simulink model "uGrid_1PH_hd_ATD_prueba"  (R2018a)
settings: Solver=ode45  StartTime=0.0  StopTime=1.5  FixedStep=1e-4  MaxStep=1e-4  RelTol=1e-3
PreLoadFcn:
  | SimulinkInit
InitFcn:
  | SimulinkInit
values from neighbouring files (symbols this model uses):
  Ad = sysd.A    [SimulinkInit.m]
  b = 4.91    [parametros_BIO.m]
  Bd = sysd.B    [SimulinkInit.m]
  C = C1+C2+C3+Cl    (= 0.002654)    [SimulinkInit.m]    (also in parametros_BIO.m = 1)
  C1 = Cd(1,:)    [SimulinkInit.m]
  C2 = Cd(2,:)    [SimulinkInit.m]
  C3 = Cd(3,:)    [SimulinkInit.m]
  C4 = Cd(4,:)    [SimulinkInit.m]
  Cd = sysd.C    [SimulinkInit.m]
  K = 25    [parametros_BIO.m]    (also in uio_linear.m = K1+E*H)
  K1 = 1.15    [SimulinkInit.m]    (also in parametros_BIO.m = 9.66; uio_linear.m = K1')
  K11 = 0.8    [parametros_BIO.m]
  K2 = 1    [SimulinkInit.m]    (also in parametros_BIO.m = 6.97)
  K22 = 0.2    [parametros_BIO.m]
  K3 = 1    [SimulinkInit.m]    (also in parametros_BIO.m = 31.8)
  K33 = 0.23    [parametros_BIO.m]
  K4 = 15.1    [parametros_BIO.m]
  Kd = 0.02    [parametros_BIO.m]
  Kdc = 0.02    [parametros_BIO.m]
  Kf = 1    [parametros_BIO.m]
  Kh = 1.2    [parametros_BIO.m]
  Ks = 21.5    [parametros_BIO.m]
  Ksc = 3    [parametros_BIO.m]
  Kv = 1    [parametros_BIO.m]
  Sbin = 13.8    [parametros_BIO.m]
  Svin = 2.91    [parametros_BIO.m]
  T1 = 0.4    [parametros_BIO.m]
  T2 = 1    [parametros_BIO.m]
  T3 = 15    [parametros_BIO.m]
  T4 = 2.5    [parametros_BIO.m]
  T5 = 3.3    [parametros_BIO.m]
  Tao1 = 0.5    [SimulinkInit.m]
  Tcd = 0.2    [parametros_BIO.m]
  Tcr = 0.01    [parametros_BIO.m]
  Tf = 0.04    [parametros_BIO.m]
  tm = 1e-4    (= 0.0001)    [SimulinkInit.m]
  Tr = 950    [parametros_BIO.m]
  Tt = 450    [parametros_BIO.m]
  Ttd = 0.04    [parametros_BIO.m]
  Tv = 0.05    [parametros_BIO.m]
  V = 20    [parametros_BIO.m]
  wref = 70000    [parametros_BIO.m]
  X_acid = 1.2    [parametros_BIO.m]
  X_meth = 0.35    [parametros_BIO.m]
  Z = 3    [parametros_BIO.m]
undefined symbols (not defined in the file or in its folder): F1, F2, F3, F4, G, GF, H1, H2, H3, H4, Ion, K1U, K2U, K3U, K4U, Lithium, ss1, ss2
libraries: powerlib x58, dsparch4 x12, truetime x12, powerlib_meascontrol x4, simulink x1, electricdrivelib x1
(part 1 of 3)
settings Model: Creator=erich  LastModifiedBy=carma
settings CodeAppCC: StateflowObjectComments=on
settings SimscapeCC: SimscapeNormalizeSystem=off

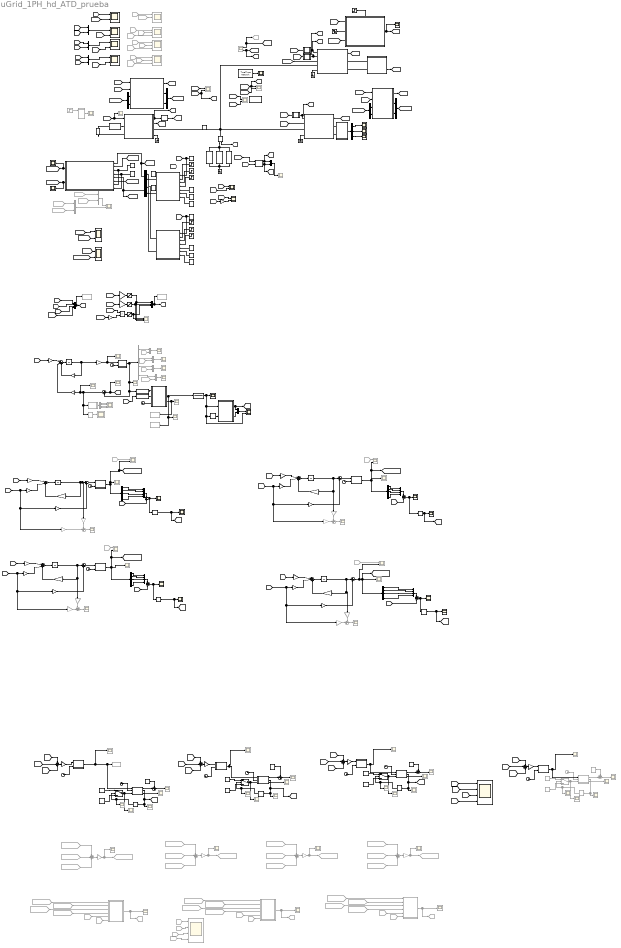
== system uGrid_1PH_hd_ATD_prueba ==
  note: DIESEL VSI
  note: Load
  note: BIO - CSI
  note: RENEWABLE - CSI
  note: Nodo De Optimizacion
  1Ph_Inverter_bio : Subsystem  mask{st_time=0, f_sw=12000, samp_f=1e-6}
      mask prompts: st_time "Tiempo muerto (Start)"; f_sw "Switching frequency"; samp_f "samplig"
      mask Display:
      | port_label('input', 1, 'd', 'texmode', 'on')
      | 
      | port_label('lconn', 1, 'DC +')
      | port_label('lconn', 2, 'DC -')
      | 
      | 
      | port_label('rconn', 1, 'V_{out+}')
      | port_label('rconn', 2, 'B_{out-}')
      | 
      | 
      | port_label('output', 1, 'I_{out}', 'texmode', 'on')
      | port_label('output', 2, 'V_{out}', 'texmode', 'on')
      | 
      | plot([0.1 .9], [0.1 .9])
      | plot([0.2 .4], [.7 .7])
      | plot([0.2 .24], [.65 .65])
      | plot([0.28 .32], [.65 .65])
      | plot([0.36 .40], [.65 .65])
      | 
      | plot([.5:.01:.7], .25+sin(30*[.2:.01:.4])/10)
  1Ph_Inverter_bio1 : Subsystem  mask{st_time=0, f_sw=12000, samp_f=1e-6}
      mask prompts: st_time "Tiempo muerto (Start)"; f_sw "Switching frequency"; samp_f "samplig"
      mask Display:
      | port_label('input', 1, 'd', 'texmode', 'on')
      | 
      | port_label('lconn', 1, 'DC +')
      | port_label('lconn', 2, 'DC -')
      | 
      | 
      | port_label('rconn', 1, 'V_{out+}')
      | port_label('rconn', 2, 'B_{out-}')
      | 
      | 
      | port_label('output', 1, 'I_{out}', 'texmode', 'on')
      | port_label('output', 2, 'V_{out}', 'texmode', 'on')
      | port_label('output', 3, 'I_{cap}', 'texmode', 'on')
      | 
      | plot([0.1 .9], [0.1 .9])
      | plot([0.2 .4], [.7 .7])
      | plot([0.2 .24], [.65 .65])
      | plot([0.28 .32], [.65 .65])
      | plot([0.36 .40], [.65 .65])
      | 
      | plot([.5:.01:.7], .25+sin(30*[.2:.01:.4])/10)
  1Ph_Inverter_diesel : Subsystem  mask{st_time=0, f_sw=12000, samp_f=1e-6}
      mask prompts: st_time "Tiempo muerto (Start)"; f_sw "Switching frequency"; samp_f "Sampling frequency"
      mask Display:
      | port_label('input', 1, 'd', 'texmode', 'on')
      | 
      | port_label('lconn', 1, 'DC +')
      | port_label('lconn', 2, 'DC -')
      | 
      | 
      | port_label('rconn', 1, 'V_{out+}')
      | port_label('rconn', 2, 'B_{out-}')
      | 
      | 
      | port_label('output', 1, 'I_{out}', 'texmode', 'on')
      | port_label('output', 2, 'V_{out}', 'texmode', 'on')
      | 
      | plot([0.1 .9], [0.1 .9])
      | plot([0.2 .4], [.7 .7])
      | plot([0.2 .24], [.65 .65])
      | plot([0.28 .32], [.65 .65])
      | plot([0.36 .40], [.65 .65])
      | 
      | plot([.5:.01:.7], .25+sin(30*[.2:.01:.4])/10)
  Bus Selector : BusSelector  OutputSignals=SOC (%),Current (A),Voltage (V)
  CSI_Control_BIO : Subsystem
  CSI_Control_DIESEL : Subsystem
  Clock{,1..5,14,18..22} (12 alike) : Clock
  Clock15 : Clock  Commented=on
  Constant : Constant  Value=1000
  Constant{1,4..5,7} (4 alike) : Constant  Value=4000
  Constant{9..11,13..14,16} (6 alike) : Constant
  Constant12 : Constant  Value=0
  Constant15 : Constant  Value=0
  Constant17 : Constant  Commented=on
  Constant18 : Constant  Commented=on  Value=0
  Constant19 : Constant  Commented=on
  Constant2 : Constant  Value=11210
  Constant3 : Constant  Value=5000
  Constant6 : Constant  Value=5000
  Constant8 : Constant  Value=0
  DC 1000V : powerlib/Electrical Sources/DC Voltage Source  Amplitude=1000  Measurements=None
  DIESEL + Rectifier System : Subsystem
  Delay2 : Delay  DelayLength=1
  Demux : Demux  Outputs=2
  Demux1 : Demux  Outputs=2
  Demux19 : Demux  Commented=on
  Demux2 : Demux  Commented=on
  Demux{5..8} (4 alike) : Demux  Outputs=5
  Derivative{,1..2,4} (4 alike) : Derivative  CoefficientInTFapproximation=0
  Derivative3 : Derivative  Commented=on  CoefficientInTFapproximation=0
  DynMat : Constant  Value=G
  DynMat_RespLibre : Constant  Value=GF
  From100 : From  Commented=on  GotoTag=x_hat_uio3
  From101 : From  Commented=on  GotoTag=x_hat_uio4
  From116 : From  Commented=on  GotoTag=x_hat_uio1
  From117 : From  Commented=on  GotoTag=rol
  From118 : From  Commented=on  GotoTag=ruo1
  From119 : From  Commented=on  GotoTag=x_hat_uio21
  From120 : From  Commented=on  GotoTag=x_hat_uio22
  From121 : From  Commented=on  GotoTag=x_hat_uio23
  From122 : From  Commented=on  GotoTag=x_hat_uio2
  From123 : From  Commented=on  GotoTag=x_hat_uio31
  From124 : From  Commented=on  GotoTag=x_hat_uio32
  From125 : From  Commented=on  GotoTag=x_hat_uio33
  From126 : From  Commented=on  GotoTag=x_hat_uio41
  From127 : From  Commented=on  GotoTag=x_hat_uio42
  From128 : From  Commented=on  GotoTag=x_hat_uio43
  From129 : From  Commented=on  GotoTag=x_hat_uio3
  From130 : From  Commented=on  GotoTag=x_hat_uio4
  From131 : From  Commented=on  GotoTag=x_hat_uio1
  From132 : From  Commented=on  GotoTag=rol
  From133 : From  Commented=on  GotoTag=ruo2
  From134 : From  Commented=on  GotoTag=x_hat_uio2
  From135 : From  Commented=on  GotoTag=x_hat_uio3
  From136 : From  Commented=on  GotoTag=x_hat_uio4
  From137 : From  Commented=on  GotoTag=x_hat_uio1
  From138 : From  Commented=on  GotoTag=rol
  From139 : From  Commented=on  GotoTag=ruo3
  From140 : From  Commented=on  GotoTag=x_hat_uio2
  From143 : From  Commented=on  GotoTag=ca4
  From144 : From  Commented=on  GotoTag=ca3
  From145 : From  Commented=on  GotoTag=ca2
  From148 : From  Commented=on  GotoTag=ca1
  From150 : From  Commented=on  GotoTag=V_vsi
  From153 : From  Commented=on  GotoTag=I3
  From154 : From  Commented=on  GotoTag=I2
  From155 : From  Commented=on  GotoTag=I1
  From159 : From  Commented=on  GotoTag=I1r
  From160 : From  Commented=on  GotoTag=I2r
  From162 : From  Commented=on  GotoTag=I3r
  From163 : From  Commented=on  GotoTag=Vlreal
  From165 : From  Commented=on  GotoTag=ruo3
  From166 : From  Commented=on  GotoTag=ruo1
  From167 : From  Commented=on  GotoTag=ruo2
  From20 : From  Commented=on  GotoTag=set_BIO
  From21 : From  Commented=on  GotoTag=set_DIESEL
  From22 : From  Commented=on  GotoTag=PQ_meas_diesel
  From23 : From  Commented=on  GotoTag=PQ_meas_bio
  From{26,58,64..65} (4 alike) : From  Commented=on  GotoTag=y_ma
  From76 : From  Commented=on  GotoTag=I1
  From77 : From  Commented=on  GotoTag=I2
  From78 : From  Commented=on  GotoTag=I3
  From79 : From  Commented=on  GotoTag=V_vsi
  From97 : From  Commented=on  GotoTag=x_hat_uio11
  From98 : From  Commented=on  GotoTag=x_hat_uio12
  From99 : From  Commented=on  GotoTag=x_hat_uio13
  Gain{,1,3,7} (4 alike) : Gain  Gain=1/3
  Gain{8..11} (4 alike) : Gain  Commented=on  Gain=1/3
  Gain2 : Gain  Gain=-1
  Gain4 : Gain  Gain=2000
  Gain5 : Gain  Gain=2
  Gain6 : Gain  Gain=2000
  Goto16 : Goto  Commented=on  GotoTag=Vlreal
  Goto24 : Goto  Commented=on  GotoTag=ca1
  Goto40 : Goto  Commented=on  GotoTag=x_hat_uio1
  Goto42 : Goto  Commented=on  GotoTag=x_hat_uio2
  Goto43 : Goto  Commented=on  GotoTag=x_hat_uio3
  Goto44 : Goto  Commented=on  GotoTag=x_hat_uio4
  Goto61 : Goto  Commented=on  GotoTag=ca2
  Goto62 : Goto  Commented=on  GotoTag=ca3
  Ground{,1..3} (4 alike) : powerlib/Elements/Ground  LConnTagsString=a
  I sens A : powerlib/Measurements/Current Measurement  PhasorSimulation=off  OutputType=Complex  PSBequivalent=0
  LinearProg : MATLAB Function  TreatAsAtomicUnit=on  SystemSampleTime=1e-3
  LinearProg1 : MATLAB Function  TreatAsAtomicUnit=on  SystemSampleTime=1e-3
  MATLAB Function : MATLAB Function  TreatAsAtomicUnit=on
  MATLAB Function1 : MATLAB Function  TreatAsAtomicUnit=on
  MATLAB Function10 : MATLAB Function  TreatAsAtomicUnit=on
  MATLAB Function11 : MATLAB Function  TreatAsAtomicUnit=on
  MATLAB Function14 : MATLAB Function  Commented=on  TreatAsAtomicUnit=on
  MATLAB Function2 : MATLAB Function  Commented=on  TreatAsAtomicUnit=on
  MATLAB Function23 : MATLAB Function  TreatAsAtomicUnit=on
  MATLAB Function24 : MATLAB Function  TreatAsAtomicUnit=on
  MATLAB Function25 : MATLAB Function  TreatAsAtomicUnit=on
  MATLAB Function3 : MATLAB Function  TreatAsAtomicUnit=on
  MATLAB Function34 : MATLAB Function  Commented=on  TreatAsAtomicUnit=on
  MATLAB Function36 : MATLAB Function  TreatAsAtomicUnit=on
  MATLAB Function38 : MATLAB Function  Commented=on  TreatAsAtomicUnit=on
  MATLAB Function39 : MATLAB Function  Commented=on  TreatAsAtomicUnit=on
  MATLAB Function4 : MATLAB Function  TreatAsAtomicUnit=on
  MATLAB Function5 : MATLAB Function  TreatAsAtomicUnit=on
  MATLAB Function6 : MATLAB Function  TreatAsAtomicUnit=on
  MATLAB Function7 : MATLAB Function  TreatAsAtomicUnit=on
  MPC Controller : Subsystem
  MeasureNode_I1 : Subsystem
  MeasureNode_I2 : Subsystem
  MeasureNode_I3 : Subsystem
  MeasureNode_I4 : Subsystem
  Memory : Memory
  Memory1 : Memory
  Memory2 : Memory
  Memory3 : Memory  Commented=on
  Mux{,1,4..6,14,26..28} (9 alike) : Mux  Inputs=2
  Mux{2..3,9..12} (6 alike) : Mux  Commented=on  Inputs=2
  Mux{8,16..19} (5 alike) : Mux
  Mux7 : Mux  Inputs=3
  P_lp_bio : Constant  Value=500
  P_lp_diesel : Constant  Value=300
  Power : powerlib_meascontrol/Measurements/Power  Freq=60  Vinit=[1, 0]  Iinit=[1, 0]  Ts=0
      settings: SourceProductName=Simscape Power Systems
  Product1 : Product
  RL : powerlib/Elements/Series RLC Branch  LConnTagsString=__new0  RConnTagsString=__new0  BranchType=R  Resistance=10  Inductance=500e-3  SetiL0=off  InitialCurrent=0  Capacitance=100e-6  Setx0=off  InitialVoltage=0  Measurements=None
  RL1 : powerlib/Elements/Series RLC Branch  LConnTagsString=__new0  RConnTagsString=__new0  BranchType=RL  Resistance=10  Inductance=5.2  SetiL0=off  InitialCurrent=0  Capacitance=100e-6  Setx0=off  InitialVoltage=0  Measurements=None
  RL2 : powerlib/Elements/Series RLC Branch  LConnTagsString=__new0  RConnTagsString=__new0  BranchType=C  Resistance=30  Inductance=500e-3  SetiL0=off  InitialCurrent=0  Capacitance=2000e-6  Setx0=off  InitialVoltage=0  Measurements=None
  Rin : powerlib/Elements/Series RLC Branch  LConnTagsString=__new0  RConnTagsString=__new0  BranchType=R  Resistance=.001  Inductance=0  SetiL0=off  InitialCurrent=0  Capacitance=0  Setx0=off  InitialVoltage=0  Measurements=None
  Saturation3 : Saturate  UpperLimit=1000  LowerLimit=-1000
  Saturation4 : Saturate  UpperLimit=1000  LowerLimit=-1000
  Saturation5 : Saturate  UpperLimit=1000  LowerLimit=-1000
  Scope{,1..3,7,85..88} (9 alike) : Scope  Commented=on  NumInputPorts=2
  Scope{5..6,9..13,41,49..50,55,64,106,111,113,115} (16 alike) : Scope
  Scope{4,8,23,31..40,45,48,51,53,57..58,60..63,67,98..99,105,107..110,112,114,118,120..138} (53 alike) : Scope  Commented=on
  Scope15 : Scope  Commented=on  NumInputPorts=4
  Scope19 : Scope  NumInputPorts=4
  Scope{24..25,27..28,42,52,59,66,73} (9 alike) : Scope  NumInputPorts=2
  Scope{30,46,56,65,68} (5 alike) : Scope  Commented=on  NumInputPorts=3
  Scope43 : Scope  Commented=on  NumInputPorts=4
  Signal Specification : SignalSpecification  Dimensions=4
  Signal Specification1 : SignalSpecification  Dimensions=4
  Sine Wave : Sin  Amplitude=170  Frequency=2*pi*60  SampleTime=0
  Step : Step  Commented=on  Time=0  After=28  SampleTime=0
  Step1 : Step  Time=0.3  Before=20000  After=5000  SampleTime=0
  Step2 : Step  Time=.6  Before=1.2  After=.4  SampleTime=0
  Step3 : Step  Before=.7  After=.7  SampleTime=0
  Step4 : Step  Time=10e-3  SampleTime=0
  Step5 : Step  Time=.3  Before=20000  After=5000  SampleTime=0
  Step6 : Step  Time=.6  Before=1.2  After=.4  SampleTime=0
  Step7 : Step  Before=.7  After=.7  SampleTime=0
  Subsystem : Subsystem
  Sum{,3,7,15} (4 alike) : Sum  Inputs=|++
  Sum{1..2,5,11} (4 alike) : Sum  Inputs=+-
  Sum10 : Sum  Inputs=|+-
  Sum{6,12,23..24} (4 alike) : Sum  Commented=on  Inputs=-+|
  Sum{4,8..9,14,16} (5 alike) : Sum  Inputs=|+++  SampleTime=tm
  Sum{50..52,56} (4 alike) : Sum  Inputs=+++
  Sum53 : Sum  Inputs=+-|
  Sum54 : Sum  Inputs=+-|
  Sum55 : Sum  Inputs=+-|
  Sum57 : Sum  Commented=on  Inputs=+-|
  Sum{58..61} (4 alike) : Sum  Commented=on  Inputs=+++
  Switch : Switch  Criteria=u2 > Threshold
  Switch1 : Switch  Criteria=u2 > Threshold
  Switch2 : Switch  Criteria=u2 > Threshold
  Switch3 : Switch  Commented=on  Criteria=u2 > Threshold
  To Workspace : ToWorkspace  Commented=on  VariableName=det1  SampleTime=1e-4
  To Workspace1 : ToWorkspace  Commented=on  VariableName=norm1  SampleTime=1e-4
  To Workspace2 : ToWorkspace  Commented=on  VariableName=y_ma  SampleTime=1e-4
  To Workspace3 : ToWorkspace  Commented=on  VariableName=u_fs  SampleTime=1e-4
  To Workspace4 : ToWorkspace  Commented=on  VariableName=dr  SaveFormat=Structure With Time  SampleTime=-1
  Transfer Fcn6 : TransferFcn  Denominator=[0.005 1]
  TrueTime Network : truetime/TrueTime Network  nwtype=CSMA/CD (Ethernet)  nwnbr=1  nnodes=10  rate=8*1e9  minsize=512  lossprob=0  seed=0  bandwidths=[0.5 0.5]  slotsize=512  schedule=[1 1 2]  memsize=80000  buftype=Common buffer  overflow=Retransmit  dynSchedule=0  miniSlotSize=0  NIT=0  QSortMode=FIFO  sync=0  irtSchedule=0  nrtLength=0  nodeGraph=0  scheduleoutput=on
  Unit Delay{1..2,6..7,10} (5 alike) : UnitDelay  SampleTime=tm
  VSI_Controller : Subsystem
  adis1 : Gain  Gain=F3  Multiplication=Matrix(K*u) (u vector)  SampleTime=tm
  adis10 : Gain  Gain=Ld'  Multiplication=Matrix(K*u) (u vector)  SampleTime=tm
  adis11 : Gain  Gain=F1  Multiplication=Matrix(K*u) (u vector)  SampleTime=tm
  adis12 : Gain  Gain=F2  Multiplication=Matrix(K*u) (u vector)  SampleTime=tm
  adis2 : Gain  Gain=F4  Multiplication=Matrix(K*u) (u vector)  SampleTime=tm
  adis7 : Gain  Gain=Ad  Multiplication=Matrix(K*u) (u vector)  SampleTime=tm
  bdis1 : Gain  Gain=T3*Bd  Multiplication=Matrix(K*u) (u vector)  SampleTime=tm
  bdis10 : Gain  Gain=T2*Bd  Multiplication=Matrix(K*u) (u vector)  SampleTime=tm
  bdis11 : Gain  Gain=K2U  Multiplication=Matrix(K*u) (u vector)  SampleTime=tm
  bdis12 : Gain  Gain=H2  Multiplication=Matrix(K*u) (u vector)  SampleTime=tm
  bdis13 : Gain  Commented=on  Gain=eye(1)-C2*H2  Multiplication=Matrix(K*u) (u vector)  SampleTime=tm
  bdis14 : Gain  Commented=on  Gain=eye(1)-C1*H1  Multiplication=Matrix(K*u) (u vector)  SampleTime=tm
  bdis15 : Gain  Commented=on  Gain=C1  Multiplication=Matrix(K*u) (u vector)  SampleTime=tm
  bdis16 : Gain  Commented=on  Gain=C2  Multiplication=Matrix(K*u) (u vector)  SampleTime=tm
  bdis17 : Gain  Gain=T4*Bd  Multiplication=Matrix(K*u) (u vector)  SampleTime=tm
  bdis18 : Gain  Gain=K4U  Multiplication=Matrix(K*u) (u vector)  SampleTime=tm
  bdis19 : Gain  Gain=H4  Multiplication=Matrix(K*u) (u vector)  SampleTime=tm
  bdis2 : Gain  Gain=K3U  Multiplication=Matrix(K*u) (u vector)  SampleTime=tm
  bdis20 : Gain  Commented=on  Gain=eye(1)-C4*H4  Multiplication=Matrix(K*u) (u vector)  SampleTime=tm
  bdis21 : Gain  Commented=on  Gain=C4  Multiplication=Matrix(K*u) (u vector)  SampleTime=tm
  bdis3 : Gain  Gain=H3  Multiplication=Matrix(K*u) (u vector)  SampleTime=tm
  bdis4 : Gain  Commented=on  Gain=eye(1)-C3*H3  Multiplication=Matrix(K*u) (u vector)  SampleTime=tm
  bdis5 : Gain  Gain=Bd  Multiplication=Matrix(K*u) (u vector)  SampleTime=tm
  bdis6 : Gain  Commented=on  Gain=C3  Multiplication=Matrix(K*u) (u vector)  SampleTime=tm
  bdis7 : Gain  Gain=T1*Bd  Multiplication=Matrix(K*u) (u vector)  SampleTime=tm
  bdis8 : Gain  Gain=K1U  Multiplication=Matrix(K*u) (u vector)  SampleTime=tm
  bdis9 : Gain  Gain=H1  Multiplication=Matrix(K*u) (u vector)  SampleTime=tm
  cdis4 : Gain  Gain=Cd  Multiplication=Matrix(K*u) (u vector)  SampleTime=tm
  generador biomasa : Subsystem  Commented=on
  powergui : powerlib/powergui  Priority=1  SimulationMode=Continuous  SampleTime=50e-6  frequency=60  Iterations=50  frequencyindice=0  Pbase=100e6  ErrMax=1e-4  UnitsV=kV  UnitsW=MW  buscounter=0  FunctionMessages=off  echomessages=off  EnableUseOfTLC=off  CurrentSourceSwitches=off  DisableSnubberDevices=off  DisableRonSwitches=off  DisableVfSwitches=off  DisplayEquations=off  SolverType=Tustin/Backward Euler (TBE)  Interpol=off  ExternalGateDelay=off  methode=off  Ts=100  x0status=blocks  SPID=off  SwTol=0  HookPort=off  RestoreLinks=warning  ResistiveCurrentMeasurement=off  Frange=[0:2:500]  Ylog=off  Xlog=on  ShowGrid=off  save=off  variable=ZData  structure=0  ZoomFFT=off  StartTime=0.0  cycles=1  DisplayStyle=1  fundamental=60  FreqAxis=off  MaxFrequency=1000  frequencyindicesteady=1  RmsSteady=1  display=off
  1000 : Constant  IOType=siggen
  wires:
  [D_bio] -> Scope4/1, 1Ph_Inverter_bio/1(A_in)
  [D_die] -> 1Ph_Inverter_diesel/1(A_in)
  [I_bio] -> [I1], Scope2/2
  [V_bio] -> Scope2/1
  [I_die] -> [I2], Scope3/1
  [V_die] -> Scope3/2
  1Ph_Inverter_bio/1(Iout) -> [I1r], MeasureNode_I2/1(in)
  1Ph_Inverter_bio/2(Vout) -> [V_bio]
  1Ph_Inverter_diesel/1(Iout) -> [I2r], MeasureNode_I1/1(in)
  1Ph_Inverter_diesel/2(Vout) -> [V_die]
  CSI_Control_BIO/1(D) -> [D_bio]
  [I_bio] -> CSI_Control_BIO/2(I_measured)
  [V_bio] -> CSI_Control_BIO/1(V_measured)
  CSI_Control_DIESEL/1(D) -> [D_die]
  [I_die] -> CSI_Control_DIESEL/2(I_measured)
  [V_die] -> CSI_Control_DIESEL/1(V_measured)
  [I_vsi] -> Scope1/1
  [I_load] -> Scope1/2
  Mux/1 -> [PQ_meas_bio]
  [MPC_U_bio] -> Demux/1
  [MPC_U_diesel] -> Demux1/1
  Mux1/1 -> [PQ_meas_diesel]
  From21/1 -> Mux2/2  "set_DIESEL"
  From20/1 -> Mux2/1  "set_BIO"
  Mux2/1 -> Scope/1
  Mux3/1 -> Scope/2
  From22/1 -> Mux3/2  "meas_DIESEL"
  From23/1 -> Mux3/1  "meas_BIO"
  CSI_Control_BIO/2(P_measure) -> Mux/1
  CSI_Control_BIO/3(Q_measure) -> Mux/2
  CSI_Control_DIESEL/2(P_measure) -> Mux1/1
  CSI_Control_DIESEL/3(Q_measure) -> Mux1/2
  Demux1/1 -> CSI_Control_DIESEL/3(P_ref)
  Demux1/2 -> CSI_Control_DIESEL/4(Q_ref)
  Demux/1 -> CSI_Control_BIO/3(P_ref)
  Demux/2 -> CSI_Control_BIO/4(Q_ref)
  DynMat_RespLibre/1 -> MPC Controller/4(GF_bio), MPC Controller/8(GF_Diesel)
  DynMat/1 -> MPC Controller/3(G_bio), MPC Controller/7(G_Diesel)
  MPC Controller/2(MPC_DIESEL_OUT) -> [MPC_U_diesel], Scope9/1
  MPC Controller/1(MPC_BIO_OUT) -> Scope5/1, [MPC_U_bio]
  [PQ_meas_bio] -> MPC Controller/2(PQ_meas_bio)
  [PQ_meas_diesel] -> MPC Controller/6(PQ_meas_Diesel)
  Constant3/1 -> LinearProg/7(P_e_alt_min)
  Constant5/1 -> LinearProg/6(PbMax)
  Step2/1 -> LinearProg/3(kb)
  Step3/1 -> LinearProg/4(kd)
  Constant1/1 -> LinearProg/5(PdMax)
  Step1/1 -> LinearProg/2(P_e_alt)
  Mux5/1 -> [set_DIESEL], MPC Controller/5(PQref_Diesel)
  Mux4/1 -> MPC Controller/1(PQref_Bio), [set_BIO]
  VSI_Controller/1(d) -> Scope6/1, [D_vsi]
  [I_vsi] -> VSI_Controller/1(Output Current)  "OutputCurrent"
  Sine Wave/1 -> VSI_Controller/2(Ref Voltage)  "Vc_ref"
  [I_cap_vsi] -> VSI_Controller/3(Capacitor Current)
  1Ph_Inverter_bio1/3(I cap) -> [I_cap_vsi]
  [D_vsi] -> 1Ph_Inverter_bio1/1(A_in)
  1Ph_Inverter_bio1/2(Vout) -> [Vlreal], MeasureNode_I3/1(in)
  [V_vsi] -> Scope7/1, Goto16/1  "v load"
  [I_vsi] -> [I3], Scope7/2
  MeasureNode_I2/1(Out) -> [I_bio]
  MeasureNode_I1/1(Out) -> [I_die]
  MeasureNode_I4/1(Out) -> [I_vsi]
  1Ph_Inverter_bio1/1(Iout) -> [I3r], MeasureNode_I4/1(in)
  I sens A/1 -> [I_load]
  MeasureNode_I3/1(Out) -> [V_vsi]
  DIESEL + Rectifier System/2(Output DC Voltage) -> [DieselE]
  Bus Selector/2 -> Scope10/1  "<Current (A)>"
  Bus Selector/1 -> Scope12/1  "<SOC (%)>"
  Bus Selector/3 -> Scope11/1  "<Voltage (V)>"
  Subsystem/1(Out1) -> Bus Selector/1
  Step4/1 -> VSI_Controller/Enable
  TrueTime Network/1 -> Scope13/1
  Power/2 -> [Q_load], Mux6/2
  [I_load] -> Power/2
  Mux6/1 -> Scope23/1
  [V_vsi] -> Power/1  "v load"
  Power/1 -> [P_load], Mux6/1
  Constant4/1 -> LinearProg1/5(QdMax)
  Step5/1 -> LinearProg1/2(Q_e_alt)
  Constant7/1 -> LinearProg1/6(QbMax)
  Step6/1 -> LinearProg1/3(kb)
  Step7/1 -> LinearProg1/4(kd)
  Constant6/1 -> LinearProg1/7(Q_e_alt_min)
  LinearProg/1(Pbo) -> Mux4/1  "bio"
  LinearProg/2(Pdo) -> Mux5/1  "die"
  LinearProg1/1(Qbo) -> Mux4/2
  LinearProg1/2(Qdo) -> Mux5/2
  [set_BIO] -> Scope24/1
  [PQ_meas_bio] -> Scope24/2
  [set_DIESEL] -> Scope25/1
  [PQ_meas_diesel] -> Scope25/2
  Constant/1 -> [P_ref], LinearProg/1(P_load)
  Constant2/1 -> [Q_ref], LinearProg1/1(Q_load)
  [P_load] -> Scope27/1
  [P_ref] -> Scope27/2
  [Q_load] -> Scope28/1
  [Q_ref] -> Gain2/1
  Gain2/1 -> Scope28/2
  Product1/1 -> Saturation5/1
  Gain5/1 -> Product1/2
  Saturation3/1 -> Scope30/3, Mux7/1
  Gain6/1 -> Saturation4/1
  [D_die] -> Gain6/1
  [DieselE] -> Gain5/1
  [D_vsi] -> Product1/1
  Saturation5/1 -> Mux7/3, Scope30/1
  Gain4/1 -> Saturation3/1
  Saturation4/1 -> Scope30/2, Mux7/2
  [D_bio] -> Gain4/1
  Mux7/1 -> To Workspace3/1, [u_fs]
  [V_vsi] -> Mux8/4
  Mux8/1 -> To Workspace2/1, [y_ma]
  [I1] -> Mux8/1
  [I2] -> Mux8/2
  [I3] -> Mux8/3
  Demux19/4 -> Scope43/4
  MATLAB Function3/1(rol) -> To Workspace/1, Scope36/1, Transfer Fcn6/1
  MATLAB Function7/2(Th_det) -> Mux14/2
  cdis4/1 -> MATLAB Function1/1(y_hat), Scope35/1
  Delay2/1 -> MATLAB Function7/2(r1)
  [y_ma] -> Signal Specification1/1
  adis10/1 -> Sum8/2
  [y_ma] -> Scope33/1, Sum10/1
  Mux14/1 -> Scope42/1
  Unit Delay6/1 -> cdis4/1, adis7/1
  From77/1 -> Mux10/2
  Demux19/2 -> Scope43/2
  Sum10/1 -> Derivative3/1, MATLAB Function2/1(r), Scope37/1, adis10/1
  MATLAB Function2/1(y) -> Demux19/1
  Mux9/1 -> Scope31/1
  Demux2/1 -> Mux9/1
  From78/1 -> Mux11/2
  Mux12/1 -> Scope34/1
  Mux11/1 -> Scope38/1
  Demux2/3 -> Mux11/1
  Clock1/1 -> MATLAB Function3/3(tiempo)
  MATLAB Function1/1(y) -> Demux2/1, Scope40/1, Sum10/2, Signal Specification/1
  Mux10/1 -> Scope32/1
  MATLAB Function7/1(rol) -> [rol], Mux14/1
  [u_fs] -> bdis5/1
  Signal Specification/1 -> MATLAB Function3/1(y_hat)
  bdis5/1 -> Sum8/1
  Demux19/3 -> Scope43/3
  Transfer Fcn6/1 -> Scope42/2, Delay2/1, MATLAB Function7/1(r), Scope41/1
  From76/1 -> Mux9/2
  Sum8/1 -> Unit Delay6/1
  Demux2/2 -> Mux10/1
  Demux2/4 -> Mux12/1
  Clock/1 -> MATLAB Function1/2(t)
  MATLAB Function3/2(norm_rd) -> To Workspace1/1, Scope39/1
  Signal Specification1/1 -> MATLAB Function3/2(y_m)
  adis7/1 -> Sum8/3
  From79/1 -> Mux12/2
  Demux19/1 -> Scope43/1
  [I1] -> bdis20/1, bdis19/1, bdis18/1
  Sum52/1 -> Gain3/1
  bdis20/1 -> Sum12/2
  Demux5/1 -> Mux16/1
  Derivative4/1 -> [druo4], Scope115/1
  Demux5/2 -> Mux16/2
  Mux18/1 -> Sum5/1
  Demux6/2 -> Mux17/2
  bdis16/1 -> Sum24/1
  Clock4/1 -> MATLAB Function24/2(t)
  bdis13/1 -> Sum24/2
  From58/1 -> Scope86/1
  Demux5/5 -> Mux16/4
  adis2/1 -> Sum9/3
  Demux7/1 -> Mux18/1
  Demux8/1 -> Mux19/1
  bdis2/1 -> Sum4/2
  Sum6/1 -> Scope60/1
  bdis14/1 -> Sum23/2
  From65/1 -> Scope88/1
  [y_ma] -> Sum5/2
  [I2] -> bdis14/1, bdis9/1, bdis8/1
  Sum3/1 -> [x_hat_uio13], Demux7/1, Scope53/1, Scope87/2
  Demux6/5 -> Mux17/4
  Mux16/1 -> Sum1/1
  Demux7/5 -> Mux18/4
  bdis1/1 -> Sum4/1
  bdis4/1 -> Sum6/2
  [u_fs] -> bdis17/1
  Sum2/1 -> Derivative1/1, Scope50/1
  Demux6/3 -> Mux17/3
  [druo1] -> Sum52/3
  bdis21/1 -> Sum12/1
  Sum12/1 -> Scope67/1
  bdis7/1 -> Sum14/1
  Unit Delay7/1 -> adis11/1, bdis15/1, Sum/1
  bdis19/1 -> Sum7/2
  Demux8/2 -> Mux19/2
  Sum4/1 -> Unit Delay1/1
  adis1/1 -> Sum4/3
  bdis17/1 -> Sum9/1
  bdis12/1 -> Sum15/2
  Demux8/5 -> Mux19/4
  [u_fs] -> bdis10/1
  bdis15/1 -> Sum23/1
  bdis11/1 -> Sum16/2
  [I3] -> bdis13/1, bdis12/1, bdis11/1
  adis11/1 -> Sum14/3
  bdis3/1 -> Sum3/2
  Sum5/1 -> Derivative2/1, Scope55/1
  [druo4] -> Sum52/2
  adis12/1 -> Sum16/3
  Sum/1 -> MATLAB Function/1(u)
  [u_fs] -> bdis1/1
  [druo3] -> Sum52/1
  Sum9/1 -> Unit Delay2/1
  [druo4] -> Sum51/1
  Unit Delay1/1 -> bdis6/1, adis1/1, Sum3/1
  Demux6/1 -> Mux17/1
  bdis18/1 -> Sum9/2
  Gain/1 -> MATLAB Function4/1(u)
  Sum11/1 -> Derivative4/1, Scope64/1
  From64/1 -> Scope87/1
  [druo2] -> Sum50/2
  Mux19/1 -> Sum11/1
  Sum23/1 -> Scope57/1
  bdis6/1 -> Sum6/1
  Sum50/1 -> Gain/1
  Sum1/1 -> Derivative/1, Scope49/1
  [druo1] -> Sum50/1
  [u_fs] -> bdis7/1
  [y_ma] -> Sum2/2
  Sum7/1 -> MATLAB Function25/1(u)
  [druo2] -> Sum51/2
  Unit Delay10/1 -> bdis16/1, adis12/1, Sum15/1
  [druo3] -> Sum51/3
  [druo3] -> Sum50/3
  Sum24/1 -> Scope58/1
  Sum51/1 -> Gain1/1
  Mux17/1 -> Sum2/1
  Sum16/1 -> Unit Delay10/1
  bdis9/1 -> Sum/2
  Sum15/1 -> MATLAB Function24/1(u)
  Clock5/1 -> MATLAB Function25/2(t)
  MATLAB Function/1(y) -> Scope51/1, [x_hat_uio11], Scope85/2, Demux5/1
  Sum14/1 -> Unit Delay7/1
  [y_ma] -> Sum11/2
  Clock3/1 -> MATLAB Function/2(t)
  Unit Delay2/1 -> bdis21/1, adis2/1, Sum7/1
  Demux7/3 -> Mux18/3
  [y_ma] -> Sum1/2
  [V_vsi] -> bdis4/1, bdis3/1, bdis2/1
  From26/1 -> Scope85/1
  Demux5/3 -> Mux16/3
  Demux8/3 -> Mux19/3
  bdis8/1 -> Sum14/2
  bdis10/1 -> Sum16/1
  Demux7/2 -> Mux18/2
  Derivative/1 -> [druo1], Scope106/1
  Derivative1/1 -> [druo2], Scope111/1
  Derivative2/1 -> [druo3], Scope113/1
  Clock2/1 -> MATLAB Function4/2(t)
  Clock18/1 -> MATLAB Function6/2(t)
  Gain1/1 -> MATLAB Function6/1(u)
  Clock19/1 -> MATLAB Function10/2(t)
  Gain3/1 -> MATLAB Function10/1(u)
  Constant11/1 -> Sum53/1
  MATLAB Function36/3(o) -> Scope123/1
  Switch/1 -> Scope122/1, MATLAB Function36/3(ban)
  Sum53/1 -> Scope120/1
  MATLAB Function36/1(r) -> Sum53/2
  MATLAB Function36/2(c) -> [ruo1], Scope121/1, Memory/1
  Clock20/1 -> MATLAB Function36/2(t)
  MATLAB Function4/1(y) -> Scope108/1, MATLAB Function36/1(dr), To Workspace4/1
  Constant8/1 -> Switch/1
  Constant9/1 -> Switch/3
  Memory/1 -> Scope124/1, Switch/2
  Memory1/1 -> Scope129/1, Switch1/2
  Clock21/1 -> MATLAB Function11/2(t)
  MATLAB Function6/1(y) -> MATLAB Function11/1(dr), Scope110/1
  MATLAB Function11/2(c) -> [ruo2], Scope126/1, Memory1/1
  MATLAB Function11/1(r) -> Sum54/2
  Switch1/1 -> Scope127/1, MATLAB Function11/3(ban)
  Sum54/1 -> Scope125/1
  Constant10/1 -> Sum54/1
  Constant13/1 -> Switch1/3
  MATLAB Function11/3(o) -> Scope128/1
  Constant12/1 -> Switch1/1
  Memory2/1 -> Scope134/1, Switch2/2
  Clock22/1 -> MATLAB Function23/2(t)
  MATLAB Function10/1(y) -> MATLAB Function23/1(dr), Scope112/1
  MATLAB Function23/2(c) -> [ruo3], Scope131/1, Memory2/1
  MATLAB Function23/1(r) -> Sum55/2
  Switch2/1 -> Scope132/1, MATLAB Function23/3(ban)
  Sum55/1 -> Scope130/1
  Constant14/1 -> Sum55/1
  Constant16/1 -> Switch2/3
  MATLAB Function23/3(o) -> Scope133/1
  Constant15/1 -> Switch2/1
  Derivative3/1 -> Scope99/1
  Sum57/1 -> Scope61/1
  Switch3/1 -> Scope98/1, MATLAB Function14/3(ban)
  MATLAB Function14/1(r) -> Sum57/2
  Constant17/1 -> Sum57/1
  MATLAB Function14/2(c) -> Scope62/1, Memory3/1
  Clock15/1 -> MATLAB Function14/2(t)
  Memory3/1 -> Scope107/1, Switch3/2
  MATLAB Function14/3(o) -> Scope105/1
  Constant19/1 -> Switch3/3
  Constant18/1 -> Switch3/1
  Clock14/1 -> MATLAB Function5/2(t)
  [druo2] -> Sum56/2
  Gain7/1 -> MATLAB Function5/1(u)
  [druo1] -> Sum56/3
  [druo4] -> Sum56/1
  Sum56/1 -> Gain7/1
  MATLAB Function5/1(y) -> MATLAB Function14/1(dr), Scope45/1
  From100/1 -> MATLAB Function39/3(x_hat3)
  From124/1 -> Sum60/2
  From133/1 -> MATLAB Function34/5(ruo1)
  From140/1 -> MATLAB Function39/2(x_hat2)
  MATLAB Function34/1(v1) -> Goto61/1, Scope136/1
  From139/1 -> MATLAB Function39/5(ruo1)
  From127/1 -> Sum61/2
  From117/1 -> MATLAB Function38/6(rol)
  MATLAB Function38/1(v1) -> Goto24/1, Scope109/1
  From130/1 -> MATLAB Function38/4(x_hat4)
  Sum58/1 -> Gain8/1
  From135/1 -> MATLAB Function34/3(x_hat3)
  From118/1 -> MATLAB Function38/5(ruo1)
  From128/1 -> Sum61/3
  From132/1 -> MATLAB Function34/6(rol)
  Gain10/1 -> Scope118/1, Goto43/1
  Sum60/1 -> Gain10/1
  From125/1 -> Sum60/3
  From137/1 -> MATLAB Function39/1(x_hat1)
  From123/1 -> Sum60/1
  From101/1 -> MATLAB Function39/4(x_hat4)
  Gain8/1 -> Scope138/1, Goto40/1
  From121/1 -> Sum59/3
  From99/1 -> Sum58/3
  From136/1 -> MATLAB Function34/4(x_hat4)
  From138/1 -> MATLAB Function39/6(rol)
  From97/1 -> Sum58/1
  From122/1 -> MATLAB Function38/2(x_hat2)
  From98/1 -> Sum58/2
  From131/1 -> MATLAB Function34/1(x_hat1)
  From129/1 -> MATLAB Function38/3(x_hat3)
  From126/1 -> Sum61/1
  From116/1 -> MATLAB Function38/1(x_hat1)
  From119/1 -> Sum59/1
  MATLAB Function39/1(v1) -> Goto62/1, Scope137/1
  Gain11/1 -> Scope135/1, Goto44/1
  Sum61/1 -> Gain11/1
  Sum59/1 -> Gain9/1
  Gain9/1 -> Scope114/1, Goto42/1
  From134/1 -> MATLAB Function34/2(x_hat2)
  From120/1 -> Sum59/2
  MATLAB Function24/1(y) -> Demux6/1, [x_hat_uio12], Scope86/2, Scope48/1
  MATLAB Function25/1(y) -> Scope63/1, [x_hat_uio21], Scope88/2, Demux8/1
  Step/1 -> generador biomasa/1(In1)
  generador biomasa/1(Vdc) -> Scope8/1
  From143/1 -> Scope15/4
  From148/1 -> Scope15/1
  From144/1 -> Scope15/3
  From145/1 -> Scope15/2
  [ruo1] -> Scope19/2
  [ruo3] -> Scope19/4
  [ruo2] -> Scope19/3
  [rol] -> Scope19/1
  [V_vsi] -> Scope73/2
  From153/1 -> Scope65/2
  From154/1 -> Scope56/2
  From155/1 -> Scope46/2
  From159/1 -> Scope46/1
  From160/1 -> Scope56/1
  From162/1 -> Scope65/1
  From163/1 -> Scope68/1
  From150/1 -> Scope68/2
  [Vlreal] -> Scope73/1
  From166/1 -> Scope46/3
  From167/1 -> Scope56/3
  From165/1 -> Scope65/3
  [I1r] -> Mux26/1
  [I1] -> Mux26/2
  Mux26/1 -> Scope52/1
  [ruo1] -> Scope52/2
  [I3r] -> Mux28/1
  [I3] -> Mux28/2
  Mux28/1 -> Scope66/1
  [I2r] -> Mux27/1
  [I2] -> Mux27/2
  Mux27/1 -> Scope59/1
  [ruo2] -> Scope59/2
  [ruo3] -> Scope66/2
  connections:
  RL/LConn1 -- I sens A/RConn1 -- RL2/LConn1 -- RL1/LConn1
  Ground/LConn1 -- RL1/RConn1 -- RL2/RConn1 -- RL/RConn1
  1Ph_Inverter_bio/RConn2 -- Ground1/LConn1
  Rin/RConn1 -- 1Ph_Inverter_bio/LConn1
  1Ph_Inverter_diesel/RConn2 -- Ground3/LConn1
  1Ph_Inverter_diesel/RConn1 -- I sens A/LConn1 -- 1Ph_Inverter_bio/RConn1 -- 1Ph_Inverter_bio1/RConn1
  1Ph_Inverter_bio1/RConn2 -- Ground2/LConn1
  Subsystem/LConn1 -- 1Ph_Inverter_diesel/LConn1
  Subsystem/LConn2 -- 1Ph_Inverter_diesel/LConn2
  DC 1000V/RConn1 -- Rin/LConn1
  DC 1000V/LConn1 -- 1Ph_Inverter_bio/LConn2
  DIESEL + Rectifier System/LConn1 -- 1Ph_Inverter_bio1/LConn1
  DIESEL + Rectifier System/LConn2 -- 1Ph_Inverter_bio1/LConn2

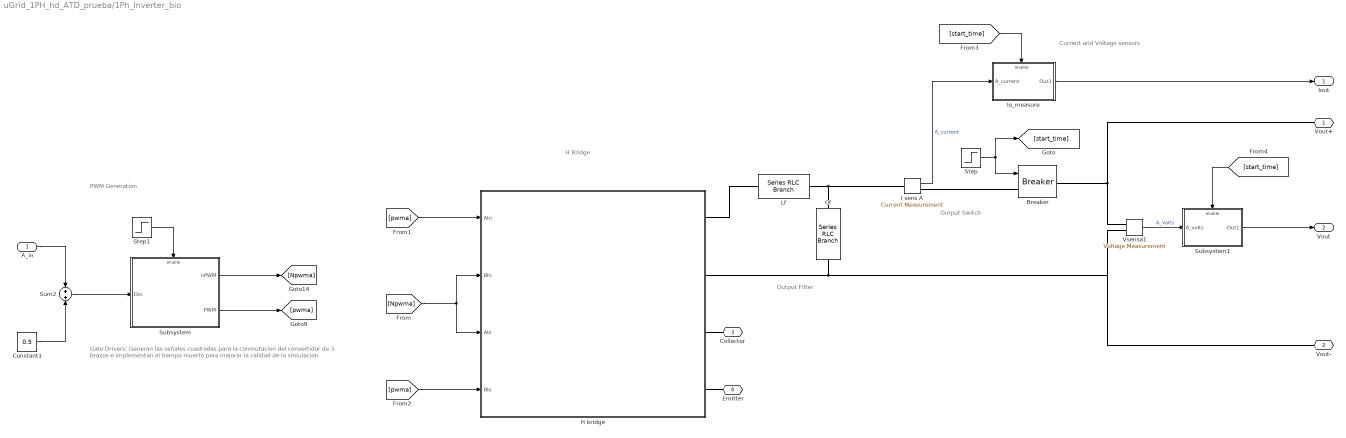
== system uGrid_1PH_hd_ATD_prueba/1Ph_Inverter_bio ==
  note: PWM Generation
  note: H Bridge
  note: Output Filter
  note: Current and Voltage sensors
  note: Output Switch
  note: Gate Drivers: Generan las señales cuadradas para
      | la conmutacion del convertidor de 3 brazos e implementan el
      | tiempo muerto para mejorar la calidad de la simulacion
  A_in : Inport
  Breaker : powerlib/Elements/Breaker  InitialState=0  SwitchingTimes="[1/60  5/60]"  External=on  BreakerResistance=0.01  SnubberResistance=1e6  SnubberCapacitance=inf  Measurements=None  MoreParameters=on  NoBreakLoop=off
      settings: SourceProductName=Simscape Power Systems
  Cf : powerlib/Elements/Series RLC Branch  LConnTagsString=__new0  RConnTagsString=__new0  BranchType=C  Resistance=1  Inductance=1e-3  SetiL0=off  InitialCurrent=0  Capacitance=22e-6  Setx0=off  InitialVoltage=0  Measurements=None
  Constant1 : Constant  Value=0.5
  H bridge : Subsystem
      mask Display:
      | port_label('input', 1, '\fontsize{12} Ahi', 'texmode', 'on')
      | port_label('input', 2, '\fontsize{12} Alo', 'texmode', 'on')
      | port_label('input', 3, '\fontsize{12} Bhi', 'texmode', 'on')
      | port_label('input', 4, '\fontsize{12} Blo', 'texmode', 'on')
      | 
      | 
      | port_label('rconn', 1, '\fontsize{12} V_{out} +', 'texmode', 'on')
      | port_label('rconn', 2, '\fontsize{12} V_{out} -', 'texmode', 'on')
      | 
      | port_label('rconn', 3, '\fontsize{12} Collector', 'texmode', 'on')
      | port_label('rconn', 4, '\fontsize{12} Emitter', 'texmode', 'on')
      | 
      | lvx = [.1 .1];
      | lvy = [.1 .2];
      | lhx = [.1 .2];
      | lhy = [.1 .1];
      | 
      | 
      | % se dibujan los interruptores de la izquierda
      | plot(lvx+.07, lvy*.8+.028+.1)
      | plot(lvx+.1, lvy+.1)
      | plot(lhx*.5+.15, lhy+.1)
      | plot(lhx*.5+.15, lhy+.2)
      | plot(lhx*.5+.07, lhy+.15)
      | 
      | d=0.5;
      | 
      | plot(lvx+.07, lvy*.8+.028+.1+d)
      | plot(lvx+.1, lvy+.1+d)
      | plot(lhx*.5+.15, lhy+.1+d)
      | plot(lhx*.5+.15, lhy+.2+d)
      | plot(lhx*.5+.07, lhy+.15+d)
      | 
      | 
      | % se dibujan los interruptores del medio
      | h=.3;
      | 
      | %plot(lvx+.07+h, lvy*.8+.028+.1)
      | %plot(lvx+.1+h, lvy+.1)
      | %plot(lhx*.5+.15+h, lhy+.1)
      | %plot(lhx*.5+.15+h, lhy+.2)
      | %plot(lhx*.5+.07+h, lhy+.15)
      | 
      | %plot(lvx+.07+h, lvy*.8+.028+.1+d)
      | %plot(lvx+.1+h, lvy+.1+d)
      | %plot(lhx*.5+.15+h, lhy+.1+d)
      | %plot(lhx*.5+.15+h, lhy+.2+d)
      | %plot(lhx*.5+.07+h, lhy+.15+d)
      | 
      | % se dibujan los interruptores de la derecha
      | h=.6
      | 
      | plot(lvx+.07+h, lvy*.8+.028+.1)
      | plot(lvx+.1+h, lvy+.1)
      | plot(lhx*.5+.15+h, lhy+.1)
      | plot(lhx*.5+.15+h, lhy+.2)
      | plot(lhx*.5+.07+h, lhy+.15)
      | 
      | plot(lvx+.07+h, lvy*.8+.028+.1+d)
      | plot(lvx+.1+h, lvy+.1+d)
      | plot(lhx*.5+.15+h, lhy+.1+d)
      | plot(lhx*.5+.15+h, lhy+.2+d)
      | plot(lhx*.5+.07+h, lhy+.15+d)
      | 
      | 
      | % se conectan los interruptores.
      | plot(lvx+.15, lvy*4-.1)
      | %plot(lvx+.15+.3, lvy*4-.1)
      | plot(lvx+.15+.6, lvy*4-.1)
      | 
      | 
      | plot(lvx+.15, lvy+.7)
      | %plot(lvx+.15+.3, lvy+.7)
      | plot(lvx+.15+.6, lvy+.7)
      | 
      | plot(lvx+.15, lvy)
      | %plot(lvx+.15+.3, lvy)
      | plot(lvx+.15+.6, lvy)
      | 
      | plot(lhx*6-.35, lhy)
      | plot(lhx*6-.35, lhy+.8)
      | 
      | % raul esteban alzate 313 515 86 11
  I sens A : powerlib/Measurements/Current Measurement  PhasorSimulation=off  OutputType=Complex  PSBequivalent=0
  Io_measure : Subsystem
  Lf : powerlib/Elements/Series RLC Branch  LConnTagsString=__new0  RConnTagsString=__new0  BranchType=RL  Resistance=.1  Inductance=40e-3  SetiL0=off  InitialCurrent=0  Capacitance=1e-6  Setx0=off  InitialVoltage=0  Measurements=None
  Step : Step  Time=st_time  SampleTime=0
  Step1 : Step  Time=st_time  SampleTime=0
  Subsystem : Subsystem
  Subsystem1 : Subsystem
  Sum2 : Sum
  Vsensa1 : powerlib/Measurements/Voltage Measurement  PhasorSimulation=off  OutputType=Complex  PSBequivalent=0
  Vout+ : PMIOPort  Side=Right
  Vout- : PMIOPort  Port=2  Side=Right
  Collector : PMIOPort  Port=3  Side=Left
  Emitter : PMIOPort  Port=4  Side=Left
  Iout : Outport
  Vout : Outport  Port=2
  wires:
  Constant1/1 -> Sum2/2
  A_in/1 -> Sum2/1
  [pwma] -> H bridge/1(Ahi)
  [Npwma] -> H bridge/2(Bhi), H bridge/3(Alo)
  [pwma] -> H bridge/4(Blo)
  Step/1 -> [start_time], Breaker/1
  Sum2/1 -> Subsystem/1(Din)
  Subsystem/1(nPWM) -> [Npwma]
  Subsystem/2(PWM) -> [pwma]
  Step1/1 -> Subsystem/Enable
  I sens A/1 -> Io_measure/1(A_current)  "A_current"
  Io_measure/1(Out1) -> Iout/1
  [start_time] -> Io_measure/Enable
  Vsensa1/1 -> Subsystem1/1(A_volts)  "A_volts"
  Subsystem1/1(Out1) -> Vout/1
  [start_time] -> Subsystem1/Enable
  connections:
  H bridge/RConn3 -- Collector/RConn1
  H bridge/RConn4 -- Emitter/RConn1
  Lf/LConn1 -- H bridge/RConn1
  H bridge/RConn2 -- Vsensa1/LConn2 -- Vout-/RConn1 -- Cf/RConn1
  Breaker/LConn1 -- I sens A/RConn1
  Breaker/RConn1 -- Vout+/RConn1 -- Vsensa1/LConn1
  Cf/LConn1 -- I sens A/LConn1 -- Lf/RConn1

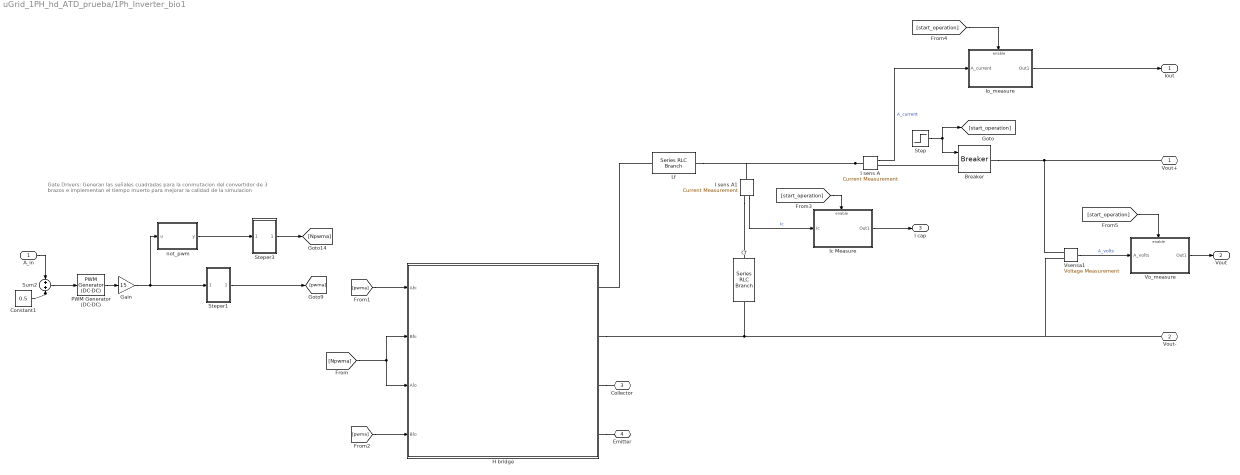
== system uGrid_1PH_hd_ATD_prueba/1Ph_Inverter_bio1 ==
  note: Gate Drivers: Generan las señales cuadradas para
      | la conmutacion del convertidor de 3 brazos e implementan el
      | tiempo muerto para mejorar la calidad de la simulacion
  A_in : Inport
  Breaker : powerlib/Elements/Breaker  InitialState=0  SwitchingTimes="[1/60  5/60]"  External=on  BreakerResistance=0.01  SnubberResistance=1e6  SnubberCapacitance=inf  Measurements=None  MoreParameters=on  NoBreakLoop=off
      settings: SourceProductName=Simscape Power Systems
  Cf : powerlib/Elements/Series RLC Branch  LConnTagsString=__new0  RConnTagsString=__new0  BranchType=C  Resistance=1  Inductance=1e-3  SetiL0=off  InitialCurrent=0  Capacitance=610e-6  Setx0=off  InitialVoltage=0  Measurements=None
  Constant1 : Constant  Value=0.5
  Gain : Gain  Gain=15
  H bridge : Subsystem
      mask Display:
      | port_label('input', 1, '\fontsize{12} Ahi', 'texmode', 'on')
      | port_label('input', 2, '\fontsize{12} Alo', 'texmode', 'on')
      | port_label('input', 3, '\fontsize{12} Bhi', 'texmode', 'on')
      | port_label('input', 4, '\fontsize{12} Blo', 'texmode', 'on')
      | 
      | 
      | port_label('rconn', 1, '\fontsize{12} V_{out} +', 'texmode', 'on')
      | port_label('rconn', 2, '\fontsize{12} V_{out} -', 'texmode', 'on')
      | 
      | port_label('rconn', 3, '\fontsize{12} Collector', 'texmode', 'on')
      | port_label('rconn', 4, '\fontsize{12} Emitter', 'texmode', 'on')
      | 
      | lvx = [.1 .1];
      | lvy = [.1 .2];
      | lhx = [.1 .2];
      | lhy = [.1 .1];
      | 
      | 
      | % se dibujan los interruptores de la izquierda
      | plot(lvx+.07, lvy*.8+.028+.1)
      | plot(lvx+.1, lvy+.1)
      | plot(lhx*.5+.15, lhy+.1)
      | plot(lhx*.5+.15, lhy+.2)
      | plot(lhx*.5+.07, lhy+.15)
      | 
      | d=0.5;
      | 
      | plot(lvx+.07, lvy*.8+.028+.1+d)
      | plot(lvx+.1, lvy+.1+d)
      | plot(lhx*.5+.15, lhy+.1+d)
      | plot(lhx*.5+.15, lhy+.2+d)
      | plot(lhx*.5+.07, lhy+.15+d)
      | 
      | 
      | % se dibujan los interruptores del medio
      | h=.3;
      | 
      | %plot(lvx+.07+h, lvy*.8+.028+.1)
      | %plot(lvx+.1+h, lvy+.1)
      | %plot(lhx*.5+.15+h, lhy+.1)
      | %plot(lhx*.5+.15+h, lhy+.2)
      | %plot(lhx*.5+.07+h, lhy+.15)
      | 
      | %plot(lvx+.07+h, lvy*.8+.028+.1+d)
      | %plot(lvx+.1+h, lvy+.1+d)
      | %plot(lhx*.5+.15+h, lhy+.1+d)
      | %plot(lhx*.5+.15+h, lhy+.2+d)
      | %plot(lhx*.5+.07+h, lhy+.15+d)
      | 
      | % se dibujan los interruptores de la derecha
      | h=.6
      | 
      | plot(lvx+.07+h, lvy*.8+.028+.1)
      | plot(lvx+.1+h, lvy+.1)
      | plot(lhx*.5+.15+h, lhy+.1)
      | plot(lhx*.5+.15+h, lhy+.2)
      | plot(lhx*.5+.07+h, lhy+.15)
      | 
      | plot(lvx+.07+h, lvy*.8+.028+.1+d)
      | plot(lvx+.1+h, lvy+.1+d)
      | plot(lhx*.5+.15+h, lhy+.1+d)
      | plot(lhx*.5+.15+h, lhy+.2+d)
      | plot(lhx*.5+.07+h, lhy+.15+d)
      | 
      | 
      | % se conectan los interruptores.
      | plot(lvx+.15, lvy*4-.1)
      | %plot(lvx+.15+.3, lvy*4-.1)
      | plot(lvx+.15+.6, lvy*4-.1)
      | 
      | 
      | plot(lvx+.15, lvy+.7)
      | %plot(lvx+.15+.3, lvy+.7)
      | plot(lvx+.15+.6, lvy+.7)
      | 
      | plot(lvx+.15, lvy)
      | %plot(lvx+.15+.3, lvy)
      | plot(lvx+.15+.6, lvy)
      | 
      | plot(lhx*6-.35, lhy)
      | plot(lhx*6-.35, lhy+.8)
      | 
      | % raul esteban alzate 313 515 86 11
  I sens A : powerlib/Measurements/Current Measurement  PhasorSimulation=off  OutputType=Complex  PSBequivalent=0
  I sens A1 : powerlib/Measurements/Current Measurement  PhasorSimulation=off  OutputType=Complex  PSBequivalent=0
  Ic Measure : Subsystem
  Io_measure : Subsystem
  Lf : powerlib/Elements/Series RLC Branch  LConnTagsString=__new0  RConnTagsString=__new0  BranchType=RL  Resistance=1e-3  Inductance=5e-3  SetiL0=off  InitialCurrent=0  Capacitance=1e-6  Setx0=off  InitialVoltage=0  Measurements=None
  PWM Generator (DC-DC) : powerlib_meascontrol/Pulse & Signal Generators/PWM Generator (DC-DC)  Fsw=f_sw  Ts=samp_f
  Step : Step  Time=st_time  SampleTime=0
  Steper1 : Subsystem
  Steper3 : Subsystem
  Sum2 : Sum
  Vo_measure : Subsystem
  Vsensa1 : powerlib/Measurements/Voltage Measurement  PhasorSimulation=off  OutputType=Complex  PSBequivalent=0
  not_pwm : MATLAB Function  TreatAsAtomicUnit=on
  Vout+ : PMIOPort  Side=Right
  Vout- : PMIOPort  Port=2  Side=Right
  Collector : PMIOPort  Port=3  Side=Left
  Emitter : PMIOPort  Port=4  Side=Left
  Iout : Outport
  Vout : Outport  Port=2
  I cap : Outport  Port=3
  wires:
  not_pwm/1(y) -> Steper3/1(In1)
  Sum2/1 -> PWM Generator (DC-DC)/1
  PWM Generator (DC-DC)/1 -> Gain/1
  Constant1/1 -> Sum2/2
  A_in/1 -> Sum2/1
  Steper1/1(Out1) -> [pwma]
  Steper3/1(Out1) -> [Npwma]
  Gain/1 -> Steper1/1(In1), not_pwm/1(u)
  [pwma] -> H bridge/1(Ahi)
  [Npwma] -> H bridge/2(Bhi), H bridge/3(Alo)
  [pwma] -> H bridge/4(Blo)
  Step/1 -> [start_operation], Breaker/1
  I sens A1/1 -> Ic Measure/1(Ic)  "Ic"
  Ic Measure/1(Out1) -> I cap/1
  [start_operation] -> Ic Measure/Enable
  Vsensa1/1 -> Vo_measure/1(A_volts)  "A_volts"
  Vo_measure/1(Out1) -> Vout/1
  I sens A/1 -> Io_measure/1(A_current)  "A_current"
  Io_measure/1(Out1) -> Iout/1
  [start_operation] -> Io_measure/Enable
  [start_operation] -> Vo_measure/Enable
  connections:
  H bridge/RConn3 -- Collector/RConn1
  H bridge/RConn4 -- Emitter/RConn1
  Lf/LConn1 -- H bridge/RConn1
  H bridge/RConn2 -- Vout-/RConn1 -- Vsensa1/LConn2 -- Cf/RConn1
  Breaker/LConn1 -- I sens A/RConn1
  Breaker/RConn1 -- Vsensa1/LConn1 -- Vout+/RConn1
  I sens A/LConn1 -- Lf/RConn1 -- I sens A1/LConn1
  I sens A1/RConn1 -- Cf/LConn1

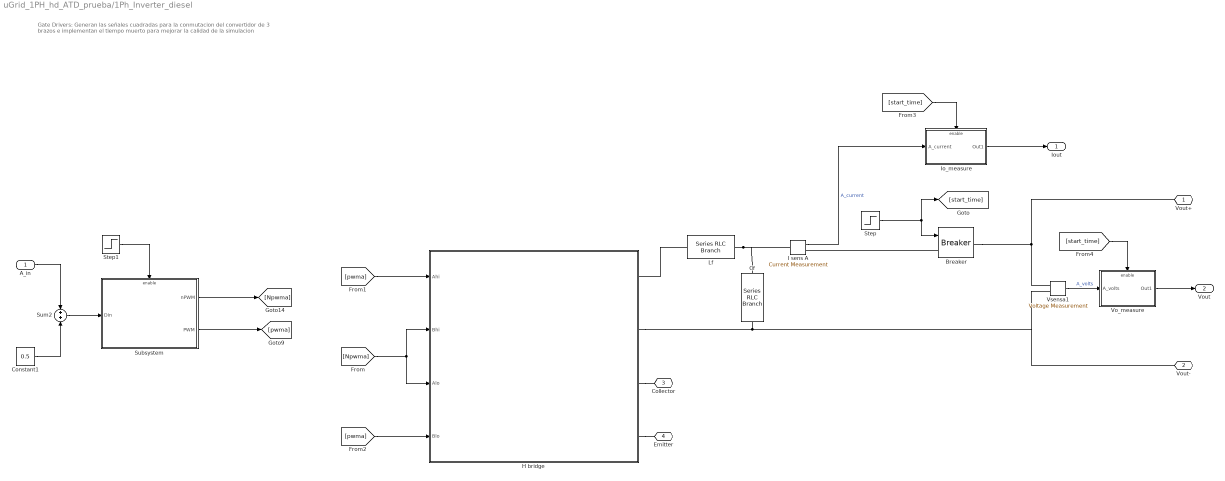
== system uGrid_1PH_hd_ATD_prueba/1Ph_Inverter_diesel ==
  note: Gate Drivers: Generan las señales cuadradas para
      | la conmutacion del convertidor de 3 brazos e implementan el
      | tiempo muerto para mejorar la calidad de la simulacion
  A_in : Inport
  Breaker : powerlib/Elements/Breaker  InitialState=0  SwitchingTimes="[1/60  5/60]"  External=on  BreakerResistance=0.01  SnubberResistance=1e6  SnubberCapacitance=inf  Measurements=None  MoreParameters=on  NoBreakLoop=off
      settings: SourceProductName=Simscape Power Systems
  Cf : powerlib/Elements/Series RLC Branch  LConnTagsString=__new0  RConnTagsString=__new0  BranchType=C  Resistance=1  Inductance=1e-3  SetiL0=off  InitialCurrent=0  Capacitance=22e-6  Setx0=off  InitialVoltage=0  Measurements=None
  Constant1 : Constant  Value=0.5
  H bridge : Subsystem
      mask Display:
      | port_label('input', 1, '\fontsize{12} Ahi', 'texmode', 'on')
      | port_label('input', 2, '\fontsize{12} Alo', 'texmode', 'on')
      | port_label('input', 3, '\fontsize{12} Bhi', 'texmode', 'on')
      | port_label('input', 4, '\fontsize{12} Blo', 'texmode', 'on')
      | 
      | 
      | port_label('rconn', 1, '\fontsize{12} V_{out} +', 'texmode', 'on')
      | port_label('rconn', 2, '\fontsize{12} V_{out} -', 'texmode', 'on')
      | 
      | port_label('rconn', 3, '\fontsize{12} Collector', 'texmode', 'on')
      | port_label('rconn', 4, '\fontsize{12} Emitter', 'texmode', 'on')
      | 
      | lvx = [.1 .1];
      | lvy = [.1 .2];
      | lhx = [.1 .2];
      | lhy = [.1 .1];
      | 
      | 
      | % se dibujan los interruptores de la izquierda
      | plot(lvx+.07, lvy*.8+.028+.1)
      | plot(lvx+.1, lvy+.1)
      | plot(lhx*.5+.15, lhy+.1)
      | plot(lhx*.5+.15, lhy+.2)
      | plot(lhx*.5+.07, lhy+.15)
      | 
      | d=0.5;
      | 
      | plot(lvx+.07, lvy*.8+.028+.1+d)
      | plot(lvx+.1, lvy+.1+d)
      | plot(lhx*.5+.15, lhy+.1+d)
      | plot(lhx*.5+.15, lhy+.2+d)
      | plot(lhx*.5+.07, lhy+.15+d)
      | 
      | 
      | % se dibujan los interruptores del medio
      | h=.3;
      | 
      | %plot(lvx+.07+h, lvy*.8+.028+.1)
      | %plot(lvx+.1+h, lvy+.1)
      | %plot(lhx*.5+.15+h, lhy+.1)
      | %plot(lhx*.5+.15+h, lhy+.2)
      | %plot(lhx*.5+.07+h, lhy+.15)
      | 
      | %plot(lvx+.07+h, lvy*.8+.028+.1+d)
      | %plot(lvx+.1+h, lvy+.1+d)
      | %plot(lhx*.5+.15+h, lhy+.1+d)
      | %plot(lhx*.5+.15+h, lhy+.2+d)
      | %plot(lhx*.5+.07+h, lhy+.15+d)
      | 
      | % se dibujan los interruptores de la derecha
      | h=.6
      | 
      | plot(lvx+.07+h, lvy*.8+.028+.1)
      | plot(lvx+.1+h, lvy+.1)
      | plot(lhx*.5+.15+h, lhy+.1)
      | plot(lhx*.5+.15+h, lhy+.2)
      | plot(lhx*.5+.07+h, lhy+.15)
      | 
      | plot(lvx+.07+h, lvy*.8+.028+.1+d)
      | plot(lvx+.1+h, lvy+.1+d)
      | plot(lhx*.5+.15+h, lhy+.1+d)
      | plot(lhx*.5+.15+h, lhy+.2+d)
      | plot(lhx*.5+.07+h, lhy+.15+d)
      | 
      | 
      | % se conectan los interruptores.
      | plot(lvx+.15, lvy*4-.1)
      | %plot(lvx+.15+.3, lvy*4-.1)
      | plot(lvx+.15+.6, lvy*4-.1)
      | 
      | 
      | plot(lvx+.15, lvy+.7)
      | %plot(lvx+.15+.3, lvy+.7)
      | plot(lvx+.15+.6, lvy+.7)
      | 
      | plot(lvx+.15, lvy)
      | %plot(lvx+.15+.3, lvy)
      | plot(lvx+.15+.6, lvy)
      | 
      | plot(lhx*6-.35, lhy)
      | plot(lhx*6-.35, lhy+.8)
      | 
      | % raul esteban alzate 313 515 86 11
  I sens A : powerlib/Measurements/Current Measurement  PhasorSimulation=off  OutputType=Complex  PSBequivalent=0
  Io_measure : Subsystem
  Lf : powerlib/Elements/Series RLC Branch  LConnTagsString=__new0  RConnTagsString=__new0  BranchType=RL  Resistance=.1  Inductance=30e-3  SetiL0=off  InitialCurrent=0  Capacitance=1e-6  Setx0=off  InitialVoltage=0  Measurements=None
  Step : Step  Time=st_time  SampleTime=0
  Step1 : Step  Time=st_time  SampleTime=0
  Subsystem : Subsystem
  Sum2 : Sum
  Vo_measure : Subsystem
  Vsensa1 : powerlib/Measurements/Voltage Measurement  PhasorSimulation=off  OutputType=Complex  PSBequivalent=0
  Vout+ : PMIOPort  Side=Right
  Vout- : PMIOPort  Port=2  Side=Right
  Collector : PMIOPort  Port=3  Side=Left
  Emitter : PMIOPort  Port=4  Side=Left
  Iout : Outport
  Vout : Outport  Port=2
  wires:
  [pwma] -> H bridge/4(Blo)
  [Npwma] -> H bridge/3(Alo), H bridge/2(Bhi)
  [pwma] -> H bridge/1(Ahi)
  A_in/1 -> Sum2/1
  Constant1/1 -> Sum2/2
  Step/1 -> [start_time], Breaker/1
  Sum2/1 -> Subsystem/1(Din)
  Subsystem/1(nPWM) -> [Npwma]
  Subsystem/2(PWM) -> [pwma]
  Step1/1 -> Subsystem/Enable
  Vsensa1/1 -> Vo_measure/1(A_volts)  "A_volts"
  Vo_measure/1(Out1) -> Vout/1
  I sens A/1 -> Io_measure/1(A_current)  "A_current"
  Io_measure/1(Out1) -> Iout/1
  [start_time] -> Io_measure/Enable
  [start_time] -> Vo_measure/Enable
  connections:
  Cf/RConn1 -- Vsensa1/LConn2 -- Vout-/RConn1 -- H bridge/RConn2
  Lf/LConn1 -- H bridge/RConn1
  H bridge/RConn4 -- Emitter/RConn1
  H bridge/RConn3 -- Collector/RConn1
  Breaker/LConn1 -- I sens A/RConn1
  Breaker/RConn1 -- Vsensa1/LConn1 -- Vout+/RConn1
  Lf/RConn1 -- I sens A/LConn1 -- Cf/LConn1

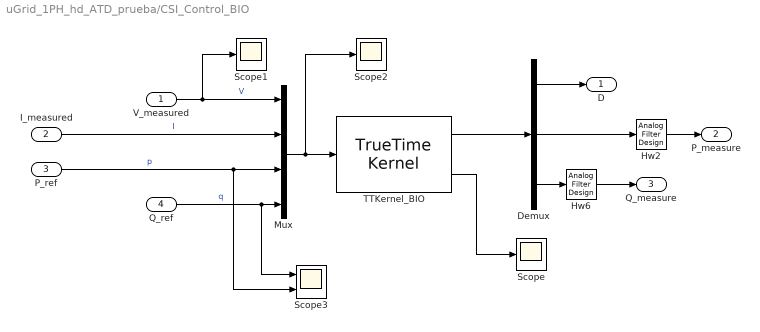
== system uGrid_1PH_hd_ATD_prueba/CSI_Control_BIO ==
  V_measured : Inport
  I_measured : Inport  Port=2
  P_ref : Inport  Port=3
  Q_ref : Inport  Port=4
  Demux : Demux  Outputs=3
  Hw2 : dsparch4/Analog Filter Design  method=Bessel  filttype=Lowpass  N=4  Wlo=30*2*pi  Whi=80  Rp=2  Rs=80
  Hw6 : dsparch4/Analog Filter Design  method=Bessel  filttype=Lowpass  N=4  Wlo=30*2*pi  Whi=80  Rp=2  Rs=80
  Mux : Mux
  Scope : Scope
  Scope1 : Scope
  Scope2 : Scope
  Scope3 : Scope  NumInputPorts=2
  TTKernel_BIO : truetime/TrueTime Kernel  sfun=BIO_init  args=1  ninputsoutputs=[4 3]  ntriggers=0  trigtype=falling  nwnodenbr=[]  clockoffsetdrift=[0 0]  schedoutput=on  battery=off  poweroutput=off
  D : Outport
  P_measure : Outport  Port=2
  Q_measure : Outport  Port=3
  wires:
  TTKernel_BIO/1 -> Demux/1
  Demux/3 -> Hw6/1
  Demux/2 -> Hw2/1
  Demux/1 -> D/1
  TTKernel_BIO/2 -> Scope/1
  Mux/1 -> Scope2/1, TTKernel_BIO/1
  V_measured/1 -> Scope1/1, Mux/1  "V"
  I_measured/1 -> Mux/2  "I"
  P_ref/1 -> Scope3/2, Mux/3  "p"
  Q_ref/1 -> Scope3/1, Mux/4  "q"
  Hw6/1 -> Q_measure/1
  Hw2/1 -> P_measure/1
